simulink library "Lib_Turbo_SFCCalc_TMATS"  (R2013b)
settings: Solver=ode45  StartTime=0.0  StopTime=10.0  RelTol=1e-3
Description:
  | Thomas Modules
settings Model: Creator=jwchapm2  LastModifiedBy=jwchapm2

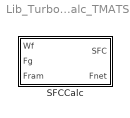
== system Lib_Turbo_SFCCalc_TMATS ==
  SFCCalc : Subsystem  mask(TMATS: SFC Calculation Library Block){}
      mask help: This block calculates specific fuel consumption (SFC) and net thrust (Fnet).

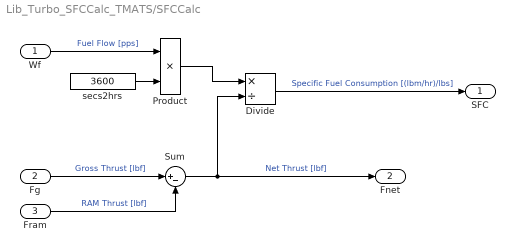
== system Lib_Turbo_SFCCalc_TMATS/SFCCalc ==
  Wf : Inport
  Fg : Inport  Port=2
  Fram : Inport  Port=3
  Divide : Product  Inputs=*/
  Product : Product
  Sum : Sum  Inputs=|+-
  secs2hrs : Constant  Value=3600
  SFC : Outport
  Fnet : Outport  Port=2
  wires:
  Fram/1 -> Sum/2  "RAM Thrust [lbf]"
  secs2hrs/1 -> Product/2
  Fg/1 -> Sum/1  "Gross Thrust [lbf]"
  Product/1 -> Divide/1
  Wf/1 -> Product/1  "Fuel Flow [pps]"
  Divide/1 -> SFC/1  "Specific Fuel Consumption [(lbm/hr)/lbs]"
  Sum/1 -> Divide/2, Fnet/1  "Net Thrust [lbf]"
